simulink model "ExperimentRobustControl"  (R2016b)
settings: Solver=ode1  StartTime=0.0  StopTime=inf  FixedStep=deltaT  RelTol=1e-3
values from neighbouring files (symbols this model uses):
  ALPHA_MAX = 15.0 * pi/180    (= 0.261799387799)    [EEN050_lab_experiment_setup.m]    (also in EEN050_lab_preparation.m)
  K_AMP = 1    [EEN050_lab_experiment_setup.m]    (also in EEN050_lab_preparation.m)
  K_CT_labb = [-71.9199164683 403.193257655 -27.8075596795 61.4313742 -3.16227766017]    [labb_LQR_controller.mat]
  K_ENC = 0    [config_srv02.m]
  K_ENC_2DIP = [-1,1].*K_ENC_2DP    [EEN050_lab_experiment_setup.m]    (also in EEN050_lab_preparation.m)
  L_CT_labb = [6.90810731192  -0.0441478085669; -0.0441478085669  16.6242650939; 23.861947831  11.0866932615; -12.1255959336  138.18406947]    [labb_LQR_controller.mat]
  OCL = 1    [EEN050_lab_preparation.m]
  qc_get_step_size = 1/1000    (= 0.001)    [EEN050_lab_experiment_setup.m]    (also in EEN050_lab_preparation.m)
  THETA_MAX = 35 * pi/180    (= 0.610865238198)    [EEN050_lab_experiment_setup.m]    (also in EEN050_lab_preparation.m)
  VMAX_AMP = 0    [config_srv02.m]
  VMAX_DAC = 10    [EEN050_lab_experiment_setup.m]    (also in EEN050_lab_preparation.m)
undefined symbols (not defined in the file or in its folder): ah, bh, ch, dh, HIL, sysc_labb
libraries: quarc_library x13, simulink_extras x1, simulink x1
settings Model: SimulationMode=external  ExtModeTrigDuration=120000  Creator=MLevis  LastModifiedBy=labb2
settings SolverCC: PositivePriorityOrder=on
settings DataIOCC: SaveFormat=StructureWithTime  SignalLoggingSaveFormat=ModelDataLogs
settings OptimizationCC: BooleanDataType=off  OptimizeBlockIOStorage=off  BufferReuse=off  GlobalBufferReuse=off  ExpressionFolding=off  ExpressionDepthLimit=2147483647  LocalBlockOutputs=off  InitFltsAndDblsToZero=on  LifeSpan=inf
settings DebuggingCC: SaveWithParameterizedLinksMsg=none  UnderspecifiedInitializationDetection=Classic  MergeDetectMultiDrivingBlocksExec=none  SignalResolutionControl=TryResolveAllWithWarning  MultiTaskDSMMsg=warning  FcnCallInpInsideContextMsg=warning  StateNameClashWarn=warning  SFUnexpectedBacktrackingDiag=warning  SFNoUnconditionalDefaultTransitionDiag=warning  SFExecutionAtInitializationDiag=none
settings HardwareCC: ProdBitPerPointer=32  ProdBitPerSizeT=32  ProdBitPerPtrDiffT=32  ProdLargestAtomicFloat=None  ProdIntDivRoundTo=Undefined  ProdEndianess=Unspecified  ProdWordSize=32  ProdHWDeviceType=32-bit Generic  TargetHWDeviceType=32-bit Generic
settings ModelReferenceCC: PropagateSignalLabelsOutOfModel=off
settings RTWCC: SystemTargetFile=quarc_win64.tlc  TemplateMakefile=quarc_default_tmf  Description=QUARC Win64 Target
settings STFCustomTargetCC: TargetPreCompLibLocation=C:\PROGRA~3\QUARC\lib\2016b\win64\release  ConcurrentExecutionCompliant=on  GeneratePreprocessorConditionals=Disable all  CPPClassGenCompliant=on  SystemTargetFile=quarc_win64.tlc
settings GRTTargetCC: TargetPreCompLibLocation=C:\PROGRA~3\QUARC\lib\2016b\win64\release  TargetLangStandard=C89/C90 (ANSI)  ParMdlRefBuildCompliant=off  CompOptLevelCompliant=off  GeneratePreprocessorConditionals=Disable all  CombineOutputUpdateFcns=off  MatFileLogging=off  GRTInterface=on  UseToolchainInfoCompliant=off  ExtMode=on  ExtModeMexFile=quarc_comm
settings ConfigComp: CovMetricSettings=dw  CovHtmlReporting=on  CovSaveCumulativeToWorkspaceVar=on  CovSaveSingleToWorkspaceVar=on  CovExternalEMLEnable=off

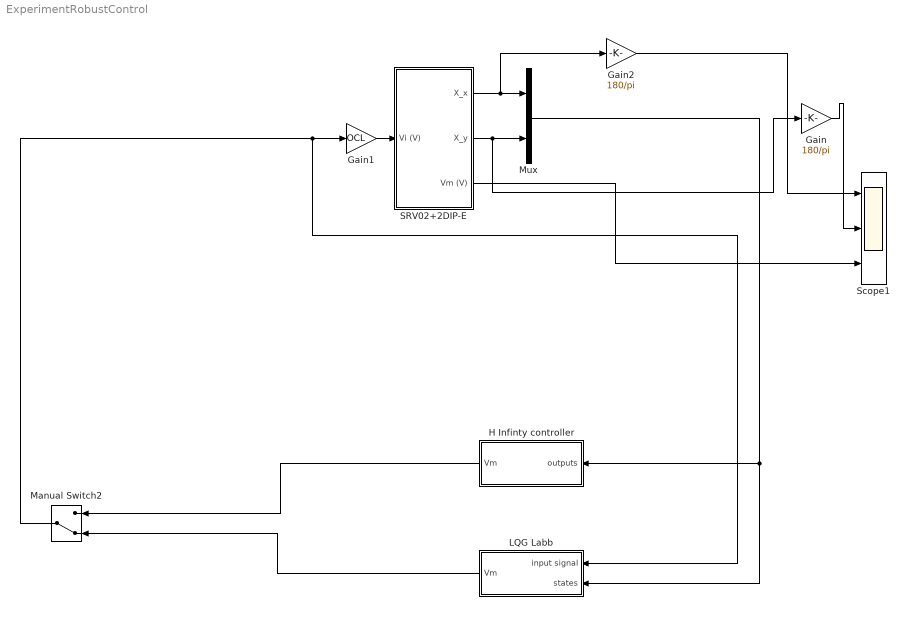
== system ExperimentRobustControl ==
  Gain : Gain  Gain=180/pi
  Gain1 : Gain  Gain=OCL
  Gain2 : Gain  Gain=180/pi
  H Infinty controller : Subsystem
  LQG Labb : Subsystem
  Manual Switch2 : ManualSwitch  CurrentSetting=0
  Mux : Mux  Inputs=2
  SRV02+2DIP-E : Subsystem
  Scope1 : Scope  NumInputPorts=3
  wires:
  SRV02+2DIP-E/2(X_y) -> Gain/1, Mux/2
  SRV02+2DIP-E/1(X_x) -> Gain2/1, Mux/1
  Mux/1 -> LQG Labb/2(states), H Infinty controller/1("outputs ")
  SRV02+2DIP-E/3(Vm (V)) -> Scope1/3
  H Infinty controller/1("Vm ") -> Manual Switch2/1
  LQG Labb/1(Vm) -> Manual Switch2/2
  Gain/1 -> Scope1/2
  Manual Switch2/1 -> LQG Labb/1(input signal), Gain1/1
  Gain2/1 -> Scope1/1
  Gain1/1 -> SRV02+2DIP-E/1(Vi (V))

== system ExperimentRobustControl/H Infinty controller ==
  "outputs " : Inport
  State-Space : StateSpace  A=ah  B=bh  C=ch  D=dh  X0=0
  "Vm " : Outport
  wires:
  State-Space/1 -> "Vm "/1
  "outputs "/1 -> State-Space/1

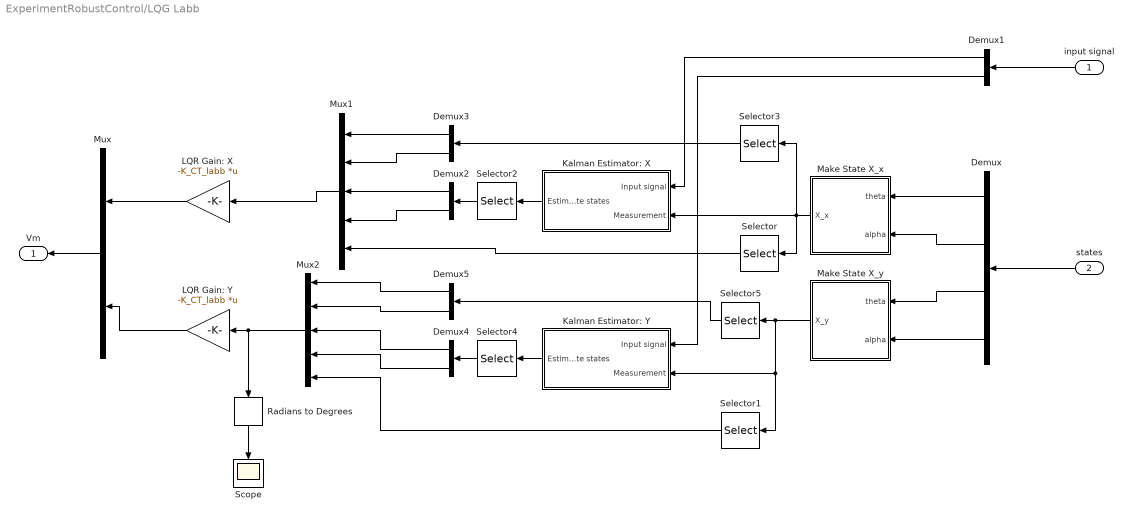
== system ExperimentRobustControl/LQG Labb ==
  input signal : Inport
  states : Inport  Port=2
  Demux : Demux
  Demux{1..5} (5 alike) : Demux  Outputs=2
  Kalman Estimator: X : Subsystem
  Kalman Estimator: Y : Subsystem
  LQR Gain: X : Gain  Gain=-K_CT_labb  Multiplication=Matrix(K*u)  SaturateOnIntegerOverflow=on  OutDataTypeStr=Inherit: Same as input  ParamDataTypeStr=Inherit: Same as input
  LQR Gain: Y : Gain  Gain=-K_CT_labb  Multiplication=Matrix(K*u)  SaturateOnIntegerOverflow=on  OutDataTypeStr=Inherit: Same as input  ParamDataTypeStr=Inherit: Same as input
  Make State X_x : Subsystem
  Make State X_y : Subsystem
  Mux : Mux  Inputs=2
  Mux1 : Mux  Inputs=5
  Mux2 : Mux  Inputs=5
  Radians to Degrees : simulink_extras/Transformations/Radians to Degrees
  Scope : Scope
  Selector : Selector  InputPortWidth=3  IndexOptions=Index vector (dialog)  Indices=[3]  OutputSizes=1
  Selector1 : Selector  InputPortWidth=3  IndexOptions=Index vector (dialog)  Indices=[3]  OutputSizes=1
  Selector2 : Selector  InputPortWidth=4  IndexOptions=Index vector (dialog)  Indices=[3 4]  OutputSizes=1
  Selector3 : Selector  InputPortWidth=3  IndexOptions=Index vector (dialog)  Indices=[1 2]  OutputSizes=1
  Selector4 : Selector  InputPortWidth=4  IndexOptions=Index vector (dialog)  Indices=[3 4]  OutputSizes=1
  Selector5 : Selector  InputPortWidth=3  IndexOptions=Index vector (dialog)  Indices=[1 2]  OutputSizes=1
  Vm : Outport
  wires:
  Mux/1 -> Vm/1
  states/1 -> Demux/1
  Demux/1 -> Make State X_x/1(theta)
  Make State X_y/1(X_y) -> Selector5/1, Selector1/1, Kalman Estimator: Y/2(Measurement)
  Demux/2 -> Make State X_x/2(alpha)
  Demux/3 -> Make State X_y/1(theta)
  Demux/4 -> Make State X_y/2(alpha)
  Demux1/1 -> Kalman Estimator: X/1(Input signal)
  Demux1/2 -> Kalman Estimator: Y/1(Input signal)
  input signal/1 -> Demux1/1
  LQR Gain: X/1 -> Mux/1
  LQR Gain: Y/1 -> Mux/2
  Make State X_x/1(X_x) -> Selector3/1, Kalman Estimator: X/2(Measurement), Selector/1
  Selector/1 -> Mux1/5
  Mux1/1 -> LQR Gain: X/1
  Kalman Estimator: X/1(Estimate states) -> Selector2/1
  Selector2/1 -> Demux2/1
  Demux2/2 -> Mux1/4
  Demux2/1 -> Mux1/3
  Demux3/1 -> Mux1/1
  Demux3/2 -> Mux1/2
  Selector3/1 -> Demux3/1
  Kalman Estimator: Y/1(Estimate states) -> Selector4/1
  Selector4/1 -> Demux4/1
  Demux4/2 -> Mux2/4
  Demux4/1 -> Mux2/3
  Demux5/1 -> Mux2/1
  Demux5/2 -> Mux2/2
  Selector5/1 -> Demux5/1
  Selector1/1 -> Mux2/5
  Radians to Degrees/1 -> Scope/1
  Mux2/1 -> Radians to Degrees/1, LQR Gain: Y/1

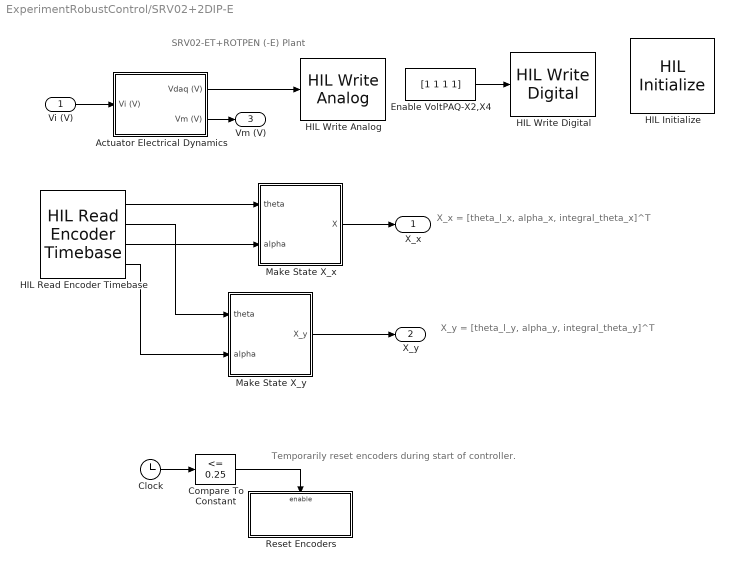
== system ExperimentRobustControl/SRV02+2DIP-E ==
  note: X_x = [theta_l_x, alpha_x, integral_theta_x]^T
  note: SRV02-ET+ROTPEN (-E) Plant
  note: X_y = [theta_l_y, alpha_y, integral_theta_y]^T
  note: Temporarily reset encoders during start of controller.
  Vi (V) : Inport
  Actuator Electrical Dynamics : Subsystem
  Clock : Clock
  Compare To Constant : simulink/Logic and Bit Operations/Compare To Constant  relop=<=  const=0.25  OutDataTypeStr=uint8  ZeroCross=off
  Enable VoltPAQ-X2,X4 : Constant  Value=[1 1 1 1]
  HIL Initialize : quarc_library/Data Acquisition/Generic/Configuration/HIL Initialize  object_name=HIL-1  board_type=q8_usb  board_number=0  board_options=update_rate=normal  exclusive=off  active=off  hardware_clocks=[0:2]  clock_modes=[]  initial_clock_frequencies=[]  set_clock_params_at_start=off  set_clock_params_at_switch_in=off  set_clock_frequencies_at_start=off  set_clock_frequencies_at_switch_in=off  analog_input_channels=[0:7]  analog_input_maximums=10  analog_input_minimums=-10  set_analog_input_params_at_start=on  set_analog_input_params_at_switch_in=off  analog_output_channels=[0:7]  analog_output_maximums=10  analog_output_minimums=-10  initial_analog_outputs=[0]  final_analog_outputs=[0]  watchdog_analog_outputs=0  set_analog_output_params_at_start=on  set_analog_output_params_at_switch_in=off  set_analog_outputs_at_start=on  set_analog_outputs_at_switch_in=off  set_analog_outputs_at_terminate=on  set_analog_outputs_at_switch_out=off  set_analog_outputs_on_watchdog=off  digital_input_channels=[]  digital_output_channels=[0:7]  digital_output_configuration=[]  initial_digital_outputs=[0]  final_digital_outputs=[0]  watchdog_digital_outputs=[0]  set_digital_output_params_at_start=off  set_digital_output_params_at_switch_in=off  set_digital_outputs_at_start=on  set_digital_outputs_at_switch_in=off  set_digital_outputs_at_terminate=on  set_digital_outputs_at_switch_out=off  set_digital_outputs_on_watchdog=off  encoder_channels=[0:7]  quadrature=[4]  encoder_filter_frequency=[]  initial_encoder_counts=[0]  set_encoder_params_at_start=on  set_encoder_params_at_switch_in=off  set_encoder_counts_at_start=on  set_encoder_counts_at_switch_in=off  pwm_channels=[0:7]  pwm_modes=0  pwm_frequency=99.532799999999995e6/4095  pwm_configuration=[0]  pwm_alignment=[0]  pwm_polarity=[1]  pwm_leading_deadband=[0]  pwm_trailing_deadband=[0]  initial_pwm_outputs=[0]  final_pwm_outputs=[0]  watchdog_pwm_outputs=[0]  set_pwm_params_at_start=on  set_pwm_params_at_switch_in=off  set_pwm_outputs_at_start=on  set_pwm_outputs_at_switch_in=off  set_pwm_outputs_at_terminate=on  set_pwm_outputs_at_switch_out=off  set_pwm_outputs_on_watchdog=off  other_output_channels=[]  initial_other_outputs=[]  final_other_outputs=[]  watchdog_other_outputs=[]  set_other_outputs_at_start=off  set_other_outputs_at_switch_in=off  set_other_outputs_at_terminate=off  set_other_outputs_at_switch_out=off  set_other_outputs_on_watchdog=off
  HIL Read Encoder Timebase : quarc_library/Data Acquisition/Generic/Timebases/HIL Read Encoder Timebase  object_name=HIL-1  clock=0  channels=0:3  samples_in_buffer=max(ceil(1/qc_get_step_size), 1)  active=on  vector_output=off  data_type_mode=Inherit via back propagation  data_type=double
  HIL Write Analog : quarc_library/Data Acquisition/Generic/Immediate I//O/HIL Write Analog  object_name=HIL-1  channels=[0,1]  sample_time=-1  active=off  vector_input=on
  HIL Write Digital : quarc_library/Data Acquisition/Generic/Immediate I//O/HIL Write Digital  object_name=HIL-1  channels=[0:3]  sample_time=-1  active=off  vector_input=on
  Make State X_x : Subsystem
  Make State X_y : Subsystem
  Reset Encoders : Subsystem  TreatAsAtomicUnit=on
  X_x : Outport  InitialOutput=0
  X_y : Outport  Port=2  InitialOutput=0
  Vm (V) : Outport  Port=3  InitialOutput=0
  wires:
  Make State X_x/1(X) -> X_x/1
  Vi (V)/1 -> Actuator Electrical Dynamics/1(Vi (V))
  Actuator Electrical Dynamics/1(Vdaq (V)) -> HIL Write Analog/1
  HIL Read Encoder Timebase/1 -> Make State X_x/1(theta)
  HIL Read Encoder Timebase/2 -> Make State X_y/1(theta)
  HIL Read Encoder Timebase/3 -> Make State X_x/2(alpha)
  HIL Read Encoder Timebase/4 -> Make State X_y/2(alpha)
  Make State X_y/1(X_y) -> X_y/1
  Clock/1 -> Compare To Constant/1
  Compare To Constant/1 -> Reset Encoders/Enable
  Actuator Electrical Dynamics/2(Vm (V)) -> Vm (V)/1
  Enable VoltPAQ-X2,X4/1 -> HIL Write Digital/1

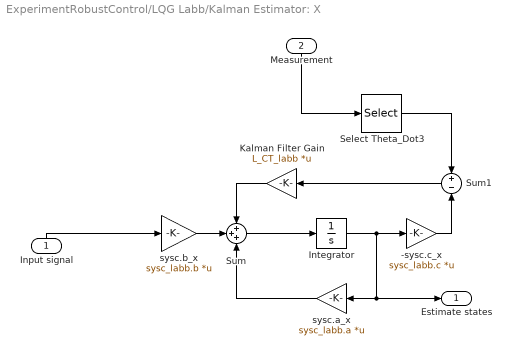
== system ExperimentRobustControl/LQG Labb/Kalman Estimator: X ==
  Input signal : Inport
  Measurement : Inport  Port=2
  -sysc.c_x : Gain  Gain=sysc_labb.c  Multiplication=Matrix(K*u) (u vector)
  Integrator : Integrator
  Kalman Filter Gain : Gain  Gain=L_CT_labb  Multiplication=Matrix(K*u) (u vector)
  Select Theta_Dot3 : Selector  InputPortWidth=3  IndexOptions=Index vector (dialog)  Indices=[1 2]  OutputSizes=1
  Sum : Sum  Inputs=+++
  Sum1 : Sum  Inputs=+|-
  sysc.a_x : Gain  Gain=sysc_labb.a  Multiplication=Matrix(K*u) (u vector)
  sysc.b_x : Gain  Gain=sysc_labb.b  Multiplication=Matrix(K*u) (u vector)
  Estimate states : Outport
  wires:
  sysc.b_x/1 -> Sum/2
  Integrator/1 -> Estimate states/1, sysc.a_x/1, -sysc.c_x/1
  Sum/1 -> Integrator/1
  Kalman Filter Gain/1 -> Sum/1
  sysc.a_x/1 -> Sum/3
  Sum1/1 -> Kalman Filter Gain/1
  -sysc.c_x/1 -> Sum1/2
  Measurement/1 -> Select Theta_Dot3/1
  Input signal/1 -> sysc.b_x/1
  Select Theta_Dot3/1 -> Sum1/1

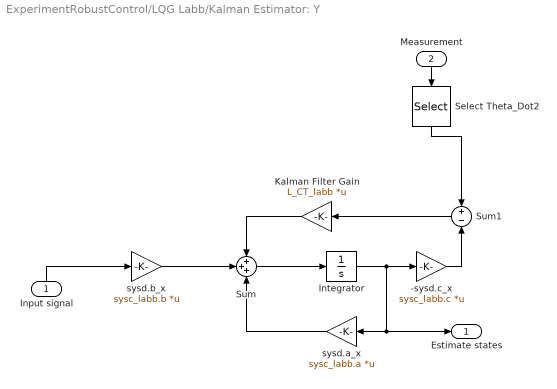
== system ExperimentRobustControl/LQG Labb/Kalman Estimator: Y ==
  Input signal : Inport
  Measurement : Inport  Port=2
  -sysd.c_x : Gain  Gain=sysc_labb.c  Multiplication=Matrix(K*u) (u vector)
  Integrator : Integrator
  Kalman Filter Gain : Gain  Gain=L_CT_labb  Multiplication=Matrix(K*u) (u vector)
  Select Theta_Dot2 : Selector  InputPortWidth=3  IndexOptions=Index vector (dialog)  Indices=[1 2]  OutputSizes=1
  Sum : Sum  Inputs=+++
  Sum1 : Sum  Inputs=+|-
  sysd.a_x : Gain  Gain=sysc_labb.a  Multiplication=Matrix(K*u) (u vector)
  sysd.b_x : Gain  Gain=sysc_labb.b  Multiplication=Matrix(K*u) (u vector)
  Estimate states : Outport
  wires:
  Measurement/1 -> Select Theta_Dot2/1
  -sysd.c_x/1 -> Sum1/2
  Sum1/1 -> Kalman Filter Gain/1
  Kalman Filter Gain/1 -> Sum/1
  Sum/1 -> Integrator/1
  Integrator/1 -> -sysd.c_x/1, sysd.a_x/1, Estimate states/1
  sysd.b_x/1 -> Sum/2
  Input signal/1 -> sysd.b_x/1
  Select Theta_Dot2/1 -> Sum1/1
  sysd.a_x/1 -> Sum/3

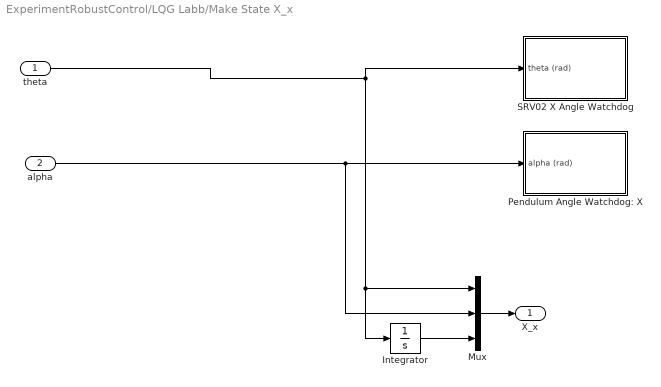
== system ExperimentRobustControl/LQG Labb/Make State X_x ==
  theta : Inport
  alpha : Inport  Port=2
  Integrator : Integrator
  Mux : Mux  Inputs=3
  Pendulum Angle Watchdog: X : Subsystem  TreatAsAtomicUnit=on
  SRV02 X Angle Watchdog : Subsystem  TreatAsAtomicUnit=on
  X_x : Outport
  wires:
  alpha/1 -> Pendulum Angle Watchdog: X/1(alpha (rad)), Mux/2
  theta/1 -> Integrator/1, Mux/1, SRV02 X Angle Watchdog/1(theta (rad))
  Mux/1 -> X_x/1
  Integrator/1 -> Mux/3

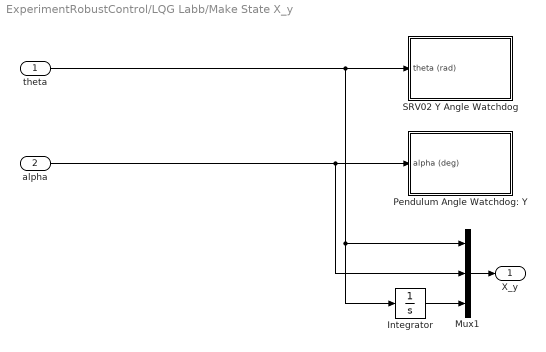
== system ExperimentRobustControl/LQG Labb/Make State X_y ==
  theta : Inport
  alpha : Inport  Port=2
  Integrator : Integrator
  Mux1 : Mux  Inputs=3
  Pendulum Angle Watchdog: Y : Subsystem  TreatAsAtomicUnit=on
  SRV02 Y Angle Watchdog : Subsystem  TreatAsAtomicUnit=on
  X_y : Outport  InitialOutput=0
  wires:
  theta/1 -> Integrator/1, Mux1/1, SRV02 Y Angle Watchdog/1(theta (rad))
  alpha/1 -> Pendulum Angle Watchdog: Y/1(alpha (deg)), Mux1/2
  Mux1/1 -> X_y/1
  Integrator/1 -> Mux1/3

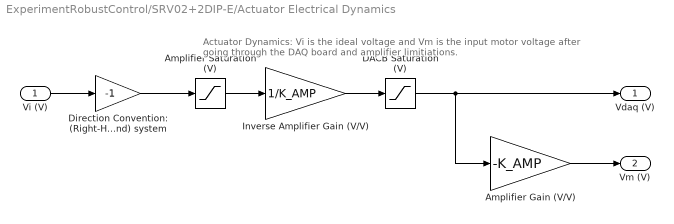
== system ExperimentRobustControl/SRV02+2DIP-E/Actuator Electrical Dynamics ==
  note: Actuator Dynamics: Vi is the ideal voltage and Vm is the
      | input motor voltage after going through the DAQ board and amplifier limitiations.
  Vi (V) : Inport
  Amplifier Gain (V/V) : Gain  Gain=-K_AMP
  Amplifier Saturation (V) : Saturate  UpperLimit=VMAX_AMP  LowerLimit=-VMAX_AMP
  DACB Saturation (V) : Saturate  UpperLimit=VMAX_DAC  LowerLimit=-VMAX_DAC
  Direction Convention: (Right-Hand) system : Gain  Gain=-1  SaturateOnIntegerOverflow=on  OutDataTypeStr=Inherit: Same as input  ParamDataTypeStr=Inherit: Same as input
  Inverse Amplifier Gain (V/V) : Gain  Gain=1/K_AMP
  Vdaq (V) : Outport
  Vm (V) : Outport  Port=2
  wires:
  Direction Convention: (Right-Hand) system/1 -> Amplifier Saturation (V)/1
  Amplifier Gain (V/V)/1 -> Vm (V)/1
  DACB Saturation (V)/1 -> Vdaq (V)/1, Amplifier Gain (V/V)/1
  Inverse Amplifier Gain (V/V)/1 -> DACB Saturation (V)/1
  Vi (V)/1 -> Direction Convention: (Right-Hand) system/1
  Amplifier Saturation (V)/1 -> Inverse Amplifier Gain (V/V)/1

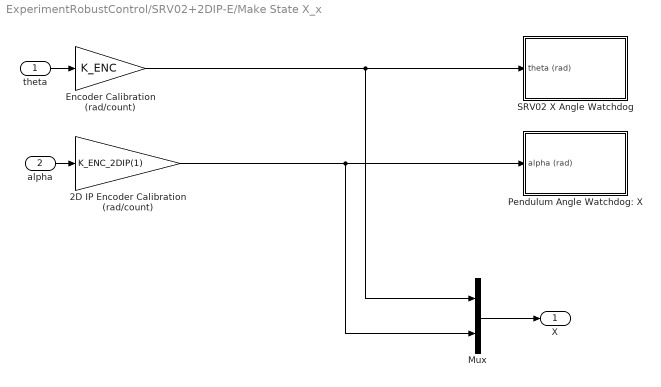
== system ExperimentRobustControl/SRV02+2DIP-E/Make State X_x ==
  theta : Inport
  alpha : Inport  Port=2
  2D IP Encoder Calibration (rad/count) : Gain  Gain=K_ENC_2DIP(1)  SaturateOnIntegerOverflow=on  OutDataTypeStr=Inherit: Same as input  ParamDataTypeStr=Inherit: Same as input
  Encoder Calibration (rad/count) : Gain  Gain=K_ENC  SaturateOnIntegerOverflow=on  OutDataTypeStr=Inherit: Same as input  ParamDataTypeStr=Inherit: Same as input
  Mux : Mux  Inputs=2
  Pendulum Angle Watchdog: X : Subsystem  TreatAsAtomicUnit=on
  SRV02 X Angle Watchdog : Subsystem  TreatAsAtomicUnit=on
  X : Outport
  wires:
  alpha/1 -> 2D IP Encoder Calibration (rad/count)/1
  theta/1 -> Encoder Calibration (rad/count)/1
  2D IP Encoder Calibration (rad/count)/1 -> Pendulum Angle Watchdog: X/1(alpha (rad)), Mux/2
  Encoder Calibration (rad/count)/1 -> Mux/1, SRV02 X Angle Watchdog/1(theta (rad))
  Mux/1 -> X/1

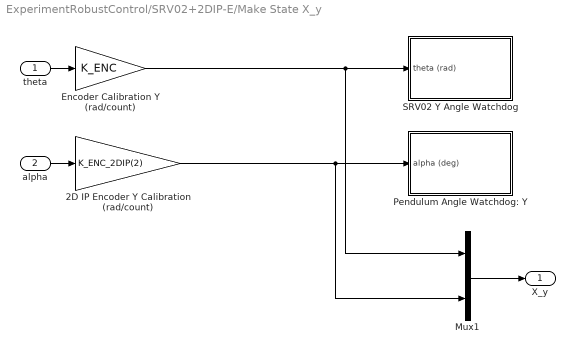
== system ExperimentRobustControl/SRV02+2DIP-E/Make State X_y ==
  theta : Inport
  alpha : Inport  Port=2
  2D IP Encoder Y Calibration (rad/count) : Gain  Gain=K_ENC_2DIP(2)  SaturateOnIntegerOverflow=on  OutDataTypeStr=Inherit: Same as input  ParamDataTypeStr=Inherit: Same as input
  Encoder Calibration Y (rad/count) : Gain  Gain=K_ENC  SaturateOnIntegerOverflow=on  OutDataTypeStr=Inherit: Same as input  ParamDataTypeStr=Inherit: Same as input
  Mux1 : Mux  Inputs=2
  Pendulum Angle Watchdog: Y : Subsystem  TreatAsAtomicUnit=on
  SRV02 Y Angle Watchdog : Subsystem  TreatAsAtomicUnit=on
  X_y : Outport  InitialOutput=0
  wires:
  Encoder Calibration Y (rad/count)/1 -> Mux1/1, SRV02 Y Angle Watchdog/1(theta (rad))
  2D IP Encoder Y Calibration (rad/count)/1 -> Pendulum Angle Watchdog: Y/1(alpha (deg)), Mux1/2
  alpha/1 -> 2D IP Encoder Y Calibration (rad/count)/1
  theta/1 -> Encoder Calibration Y (rad/count)/1
  Mux1/1 -> X_y/1

== system ExperimentRobustControl/SRV02+2DIP-E/Reset Encoders ==
  Enable : EnablePort
  HIL Set Encoder Counts : quarc_library/Data Acquisition/Generic/Configuration/HIL Set Encoder Counts  object_name=HIL-1  channels=[0:3]  source=internal  counts=0  sample_time=qc_get_step_size  active=on  vector_input=off
      settings: AttributesFormatString=(%<object_name>)

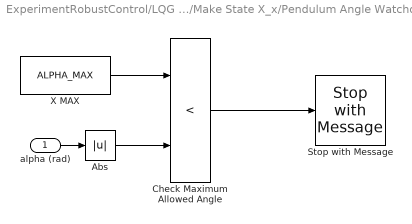
== system ExperimentRobustControl/LQG Labb/Make State X_x/Pendulum Angle Watchdog: X ==
  alpha (rad) : Inport
  Abs : Abs
  Check Maximum Allowed Angle : RelationalOperator  Operator=<  RndMeth=Nearest  InputSameDT=on
  Stop with Message : quarc_library/Sinks/Error Handling/Stop with Message  message_type=Fixed error message  message_icon=Error  message=Maximum angle reached: pendulum x angle.
  X MAX : Constant  Value=ALPHA_MAX
  wires:
  Abs/1 -> Check Maximum Allowed Angle/2
  Check Maximum Allowed Angle/1 -> Stop with Message/1
  alpha (rad)/1 -> Abs/1
  X MAX/1 -> Check Maximum Allowed Angle/1

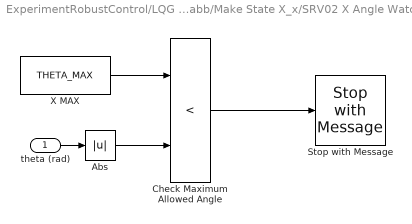
== system ExperimentRobustControl/LQG Labb/Make State X_x/SRV02 X Angle Watchdog ==
  theta (rad) : Inport
  Abs : Abs
  Check Maximum Allowed Angle : RelationalOperator  Operator=<  RndMeth=Nearest  InputSameDT=on
  Stop with Message : quarc_library/Sinks/Error Handling/Stop with Message  message_type=Fixed error message  message_icon=Error  message=Maximum angle reached: SRV02 X angle.
  X MAX : Constant  Value=THETA_MAX
  wires:
  X MAX/1 -> Check Maximum Allowed Angle/1
  theta (rad)/1 -> Abs/1
  Check Maximum Allowed Angle/1 -> Stop with Message/1
  Abs/1 -> Check Maximum Allowed Angle/2

== system ExperimentRobustControl/LQG Labb/Make State X_y/Pendulum Angle Watchdog: Y ==
  alpha (deg) : Inport
  Abs : Abs
  Check Maximum Allowed Angle : RelationalOperator  Operator=<  RndMeth=Nearest  InputSameDT=on
  Stop with Message : quarc_library/Sinks/Error Handling/Stop with Message  message_type=Fixed error message  message_icon=Error  message=Maximum angle reached: pendulum y angle.
  X MAX : Constant  Value=ALPHA_MAX
  wires:
  Abs/1 -> Check Maximum Allowed Angle/2
  Check Maximum Allowed Angle/1 -> Stop with Message/1
  alpha (deg)/1 -> Abs/1
  X MAX/1 -> Check Maximum Allowed Angle/1

== system ExperimentRobustControl/LQG Labb/Make State X_y/SRV02 Y Angle Watchdog ==
  theta (rad) : Inport
  Abs : Abs
  Check Maximum Allowed Angle : RelationalOperator  Operator=<  RndMeth=Nearest  InputSameDT=on
  Stop with Message : quarc_library/Sinks/Error Handling/Stop with Message  message_type=Fixed error message  message_icon=Error  message=Maximum angle reached: SRV02 Y angle.
  X MAX : Constant  Value=THETA_MAX
  wires:
  Abs/1 -> Check Maximum Allowed Angle/2
  Check Maximum Allowed Angle/1 -> Stop with Message/1
  theta (rad)/1 -> Abs/1
  X MAX/1 -> Check Maximum Allowed Angle/1

== system ExperimentRobustControl/SRV02+2DIP-E/Make State X_x/Pendulum Angle Watchdog: X ==
  alpha (rad) : Inport
  Abs : Abs
  Check Maximum Allowed Angle : RelationalOperator  Operator=<  RndMeth=Nearest  InputSameDT=on
  Stop with Message : quarc_library/Sinks/Error Handling/Stop with Message  message_type=Fixed error message  message_icon=Error  message=Maximum angle reached: pendulum x angle.
  X MAX : Constant  Value=ALPHA_MAX
  wires:
  Abs/1 -> Check Maximum Allowed Angle/2
  Check Maximum Allowed Angle/1 -> Stop with Message/1
  alpha (rad)/1 -> Abs/1
  X MAX/1 -> Check Maximum Allowed Angle/1

== system ExperimentRobustControl/SRV02+2DIP-E/Make State X_x/SRV02 X Angle Watchdog ==
  theta (rad) : Inport
  Abs : Abs
  Check Maximum Allowed Angle : RelationalOperator  Operator=<  RndMeth=Nearest  InputSameDT=on
  Stop with Message : quarc_library/Sinks/Error Handling/Stop with Message  message_type=Fixed error message  message_icon=Error  message=Maximum angle reached: SRV02 X angle.
  X MAX : Constant  Value=THETA_MAX
  wires:
  X MAX/1 -> Check Maximum Allowed Angle/1
  theta (rad)/1 -> Abs/1
  Check Maximum Allowed Angle/1 -> Stop with Message/1
  Abs/1 -> Check Maximum Allowed Angle/2

== system ExperimentRobustControl/SRV02+2DIP-E/Make State X_y/Pendulum Angle Watchdog: Y ==
  alpha (deg) : Inport
  Abs : Abs
  Check Maximum Allowed Angle : RelationalOperator  Operator=<  RndMeth=Nearest  InputSameDT=on
  Stop with Message : quarc_library/Sinks/Error Handling/Stop with Message  message_type=Fixed error message  message_icon=Error  message=Maximum angle reached: pendulum y angle.
  X MAX : Constant  Value=ALPHA_MAX
  wires:
  Abs/1 -> Check Maximum Allowed Angle/2
  Check Maximum Allowed Angle/1 -> Stop with Message/1
  alpha (deg)/1 -> Abs/1
  X MAX/1 -> Check Maximum Allowed Angle/1

== system ExperimentRobustControl/SRV02+2DIP-E/Make State X_y/SRV02 Y Angle Watchdog ==
  theta (rad) : Inport
  Abs : Abs
  Check Maximum Allowed Angle : RelationalOperator  Operator=<  RndMeth=Nearest  InputSameDT=on
  Stop with Message : quarc_library/Sinks/Error Handling/Stop with Message  message_type=Fixed error message  message_icon=Error  message=Maximum angle reached: SRV02 Y angle.
  X MAX : Constant  Value=THETA_MAX
  wires:
  Abs/1 -> Check Maximum Allowed Angle/2
  Check Maximum Allowed Angle/1 -> Stop with Message/1
  theta (rad)/1 -> Abs/1
  X MAX/1 -> Check Maximum Allowed Angle/1
